simulink model "nonlinear_balsa_v3"  (Simulink 7.8)
settings: Solver=ode45  StartTime=0  StopTime=10  FixedStep=dt_sim  RelTol=1e-6
undefined symbols (not defined in the file): geo, X0
libraries: vrlib x2, dspmtrx3 x1
settings Model: Creator=vickTJ  LastModifiedBy=Dan  BufferReuse=off
settings SolverCC: MaxConsecutiveMinStep=3
settings DataIOCC: ExternalInput=[0 0.571613372420885 7.40569399414751 7.40569021323198 0.00019476436772123 0.000191911234858188]  InitialState=[]  LimitDataPoints=off  MaxDataPoints=5000  SaveState=on  SignalLogging=off  DSMLogging=off  StateSaveName=stout
settings OptimizationCC: InlineParams=on  BufferReuse=off
settings DebuggingCC: UnderspecifiedInitializationDetection=Simplified  SolverPrmCheckMsg=none  FcnCallInpInsideContextMsg=Use local settings  UnconnectedInputMsg=none  UnconnectedOutputMsg=none  InitInArrayFormatMsg=none  SFInvalidInputDataAccessInChartInitDiag=none

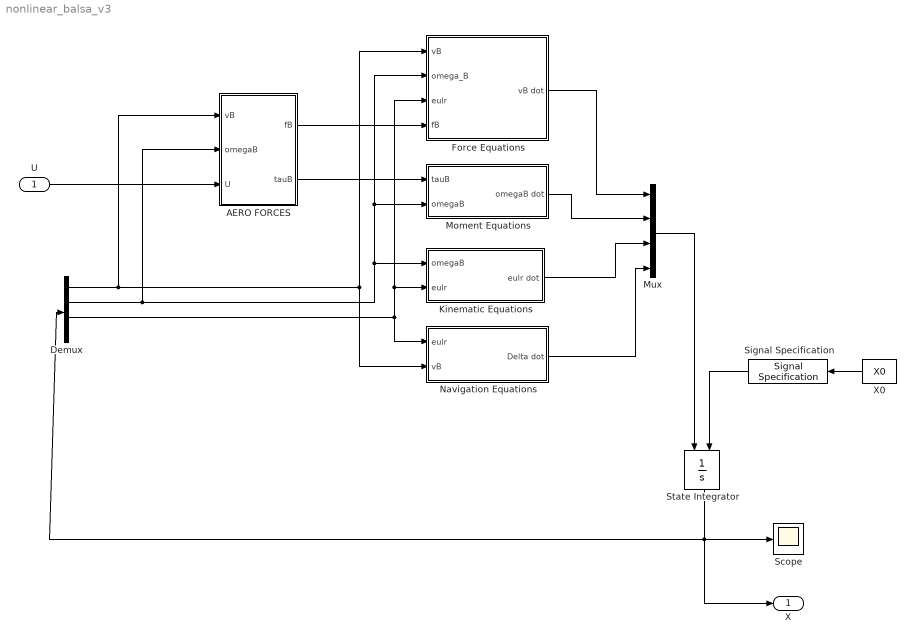
== system nonlinear_balsa_v3 ==
  U : Inport
  AERO FORCES : Subsystem
  Demux : Demux  Outputs=[3,3,3,3]
  Force Equations : Subsystem
  Kinematic Equations : Subsystem
  Moment Equations : Subsystem
  Mux : Mux  Inputs=[3,3,3,3]
  Navigation Equations : Subsystem
  Scope : Scope
  Signal Specification : SignalSpecification  Dimensions=[12,1]
  State Integrator : Integrator  InitialConditionSource=external
  X0 : Constant  Value=X0
  X : Outport
  wires:
  X0/1 -> Signal Specification/1
  Navigation Equations/1(Delta dot) -> Mux/4
  Kinematic Equations/1(eulr dot) -> Mux/3
  Mux/1 -> State Integrator/1
  State Integrator/1 -> Demux/1, Scope/1, X/1
  Force Equations/1(vB dot) -> Mux/1
  Moment Equations/1(omegaB dot) -> Mux/2
  Demux/1 -> Force Equations/1(vB), Navigation Equations/2(vB), AERO FORCES/1(vB)
  Demux/2 -> Force Equations/2(omega_B), Moment Equations/2(omegaB), Kinematic Equations/1(omegaB), AERO FORCES/2(omegaB)
  Demux/3 -> Force Equations/3(eulr), Kinematic Equations/2(eulr), Navigation Equations/1(eulr)
  AERO FORCES/1(fB) -> Force Equations/4(fB)
  AERO FORCES/2(tauB) -> Moment Equations/1(tauB)
  Signal Specification/1 -> State Integrator/2
  U/1 -> AERO FORCES/3(U)

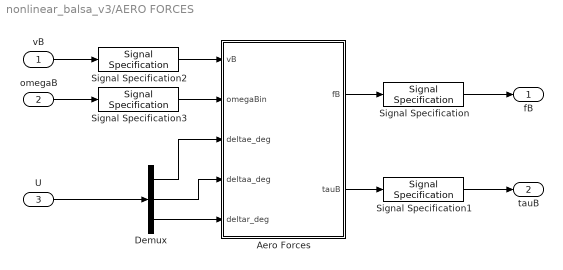
== system nonlinear_balsa_v3/AERO FORCES ==
  vB : Inport
  omegaB : Inport  Port=2
  U : Inport  Port=3
  Aero Forces : MATLAB Function  TreatAsAtomicUnit=on
  Demux : Demux  Outputs=3
  Signal Specification{,1..3} (4 alike) : SignalSpecification  Dimensions=[3,1]
  fB : Outport
  tauB : Outport  Port=2
  wires:
  Aero Forces/1(fB) -> Signal Specification/1
  Aero Forces/2(tauB) -> Signal Specification1/1
  Signal Specification/1 -> fB/1
  Signal Specification1/1 -> tauB/1
  vB/1 -> Signal Specification2/1
  omegaB/1 -> Signal Specification3/1
  Signal Specification2/1 -> Aero Forces/1(vB)
  Signal Specification3/1 -> Aero Forces/2(omegaBin)
  Demux/1 -> Aero Forces/3(deltae_deg)
  Demux/2 -> Aero Forces/4(deltaa_deg)
  Demux/3 -> Aero Forces/5(deltar_deg)
  U/1 -> Demux/1

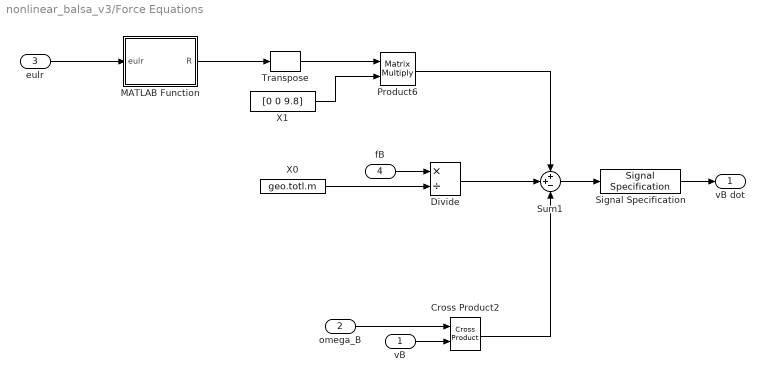
== system nonlinear_balsa_v3/Force Equations ==
  vB : Inport
  omega_B : Inport  Port=2
  eulr : Inport  Port=3
  fB : Inport  Port=4
  Cross Product2 : vrlib/Utilities/Cross Product
  Divide : Product  Inputs=*/
  MATLAB Function : MATLAB Function  TreatAsAtomicUnit=on
  Product6 : Product  Multiplication=Matrix(*)  RndMeth=Zero
  Signal Specification : SignalSpecification  Dimensions=[3,1]
  Sum1 : Sum  Inputs=++-
  Transpose : dspmtrx3/Transpose  Hermitian=off  overflowFlag=off
  X0 : Constant  Value=geo.totl.m
  X1 : Constant  Value=[0 0 9.8]
  vB dot : Outport
  wires:
  omega_B/1 -> Cross Product2/1
  Sum1/1 -> Signal Specification/1
  vB/1 -> Cross Product2/2
  Transpose/1 -> Product6/1
  X1/1 -> Product6/2
  Product6/1 -> Sum1/1
  Cross Product2/1 -> Sum1/3
  Divide/1 -> Sum1/2
  fB/1 -> Divide/1
  X0/1 -> Divide/2
  eulr/1 -> MATLAB Function/1(eulr)
  MATLAB Function/1(R) -> Transpose/1
  Signal Specification/1 -> vB dot/1

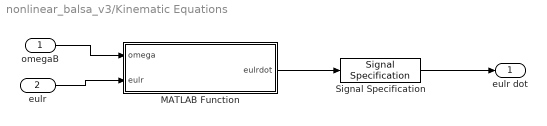
== system nonlinear_balsa_v3/Kinematic Equations ==
  omegaB : Inport
  eulr : Inport  Port=2
  MATLAB Function : MATLAB Function  TreatAsAtomicUnit=on
  Signal Specification : SignalSpecification  Dimensions=[3,1]
  eulr dot : Outport
  wires:
  omegaB/1 -> MATLAB Function/1(omega)
  eulr/1 -> MATLAB Function/2(eulr)
  MATLAB Function/1(eulrdot) -> Signal Specification/1
  Signal Specification/1 -> eulr dot/1

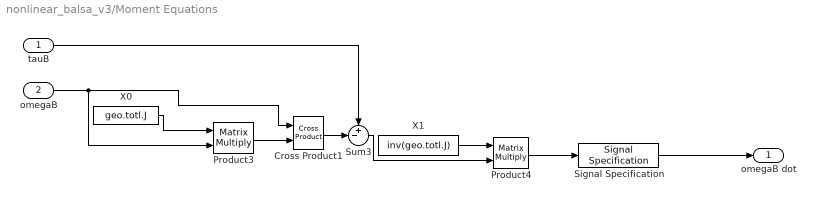
== system nonlinear_balsa_v3/Moment Equations ==
  tauB : Inport
  omegaB : Inport  Port=2
  Cross Product1 : vrlib/Utilities/Cross Product
  Product3 : Product  Multiplication=Matrix(*)  RndMeth=Zero
  Product4 : Product  Multiplication=Matrix(*)  RndMeth=Zero
  Signal Specification : SignalSpecification  Dimensions=[3,1]
  Sum3 : Sum  Inputs=+-|
  X0 : Constant  Value=geo.totl.J
  X1 : Constant  Value=inv(geo.totl.J)
  omegaB dot : Outport
  wires:
  Product4/1 -> Signal Specification/1
  X0/1 -> Product3/1
  omegaB/1 -> Product3/2, Cross Product1/1
  tauB/1 -> Sum3/1
  Cross Product1/1 -> Sum3/2
  Sum3/1 -> Product4/2
  Product3/1 -> Cross Product1/2
  X1/1 -> Product4/1
  Signal Specification/1 -> omegaB dot/1

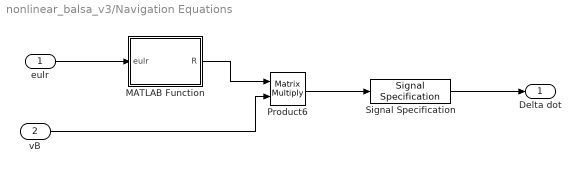
== system nonlinear_balsa_v3/Navigation Equations ==
  eulr : Inport
  vB : Inport  Port=2
  MATLAB Function : MATLAB Function  TreatAsAtomicUnit=on
  Product6 : Product  Multiplication=Matrix(*)  RndMeth=Zero
  Signal Specification : SignalSpecification  Dimensions=[3,1]
  Delta dot : Outport
  wires:
  eulr/1 -> MATLAB Function/1(eulr)
  MATLAB Function/1(R) -> Product6/1
  vB/1 -> Product6/2
  Product6/1 -> Signal Specification/1
  Signal Specification/1 -> Delta dot/1

== matlab function Force Equations/MATLAB Function ==
  data: eulr input double; R output double
function R =eulr2R(eulr)
    phi=eulr(1);
    theta=eulr(2);
    psi=eulr(3);
    R=[cos(psi)*cos(theta), cos(psi)*sin(phi)*sin(theta)-cos(phi)*sin(psi), sin(phi)*sin(psi)+cos(phi)*cos(psi)*sin(theta);
        cos(theta)*sin(psi), cos(phi)*cos(psi)+sin(phi)*sin(psi)*sin(theta), cos(phi)*sin(psi)*sin(theta)-cos(psi)*sin(phi);
        -sin(theta), cos(theta)*sin(phi), cos(phi)*cos(theta)];
end

== matlab function Kinematic Equations/MATLAB Function ==
  data: omega input double; eulr input double; eulrdot output double
function eulrdot=omega2eulrdot(omega,eulr)
    p=omega(1);
    q=omega(2);
    r=omega(3);
    phi=eulr(1);
    theta=eulr(2);
    psi=eulr(3);
    eulrdot=[1 tan(theta)*sin(phi) tan(theta)*cos(phi); 0 cos(phi) -sin(phi); 0 sin(phi)/cos(theta) cos(phi)/cos(theta)]*[p; q; r];
end

== matlab function Navigation Equations/MATLAB Function ==
  data: eulr input double; R output double
function R =eulr2R(eulr)
    phi=eulr(1);
    theta=eulr(2);
    psi=eulr(3);
    R=[cos(psi)*cos(theta), cos(psi)*sin(phi)*sin(theta)-cos(phi)*sin(psi), sin(phi)*sin(psi)+cos(phi)*cos(psi)*sin(theta);
        cos(theta)*sin(psi), cos(phi)*cos(psi)+sin(phi)*sin(psi)*sin(theta), cos(phi)*sin(psi)*sin(theta)-cos(psi)*sin(phi);
        -sin(theta), cos(theta)*sin(phi), cos(phi)*cos(theta)];
end

== matlab function AERO FORCES/Aero Forces ==
  data: fB output double; tauB output double; vB input double; omegaBin input double; deltae_deg input double; deltaa_deg input double; deltar_deg input double
function [fB,tauB]=aero_forces_v1(vB,omegaBin,deltae_deg,deltaa_deg,deltar_deg)

[m,n]=size(omegaBin);
if m==n %if input is square, skew-symmetric matrix: calculate output vector
    omegaB=[0.5*(omegaBin(3,2)-omegaBin(2,3)), 0.5*(-omegaBin(3,1)+omegaBin(1,3)), 0.5*(omegaBin(2,1)-omegaBin(1,2))];
else
    omegaB=[0 -omegaBin(3) omegaBin(2); omegaBin(3) 0 -omegaBin(1); -omegaBin(2) omegaBin(1) 0];

% vB=vB*2;
% omegaB=omegaB*2;
% xihatB=[[0 -0.2948 0.5520; 0.2948 0 0.0009; -0.5520 -0.0009 0] [1; 1; 1]; zeros(1,4)];

xihatB=[omegaB [vB(1); vB(2); vB(3)]; zeros(1,4)];

%%%%%%%%%%%%%%%%%%%%%%%%%%%%%%%%%%%%%%%%%%%%%%%%%%%%%%%%%%%%%%%%%%%%%%%%%%%
%Control surface deflections in radians
aer.delt.e=deltae_deg*pi/180;
aer.delt.a=deltaa_deg*pi/180;
aer.delt.r=deltar_deg*pi/180;

vel.totl=[xihatB(1,4) xihatB(2,4) xihatB(3,4)];
vel.u=vel.totl(1);
vel.v=vel.totl(2);
vel.w=vel.totl(3);
vel.omega=hat(xihatB(1:3,1:3));
vel.p=vel.omega(1);
vel.q=vel.omega(2);
vel.r=vel.omega(3);
vel.VT=norm(vel.totl);
vel.alpha=atan2(vel.w,vel.u); 
vel.beta=asin(vel.v/vel.VT);

%%%%%%%%%%%%%%%%%%%%%%%%%%%%%%%%%%%%%%%%%%%%%%%%%%%%%%%%%%%%%%%%%%%%%%%%%%%
%LONGITUDINAL DYNAMICS
%Calculate effective uvw velocity components at wing (in body axes, NOT including surface deflections)
vel.wing.totl=vel.totl+cross(vel.omega,XYZ.wing.rqc);
vel.wing.u=vel.wing.totl(1);
vel.wing.v=vel.wing.totl(2);
vel.wing.w=vel.wing.totl(3);
vel.wing.VT=norm(vel.wing.totl);
vel.wing.alpha=atan2(vel.wing.w,vel.wing.u); 
vel.wing.beta=asin(vel.wing.v/vel.wing.VT);

%Calculate effective uvw velocity components at horizontal tail (in body axes, including surface deflections)
vel.htai.totl=vel.totl+cross(vel.omega,XYZ.htai.rqc);
vel.htai.u=vel.htai.totl(1);
vel.htai.v=vel.htai.totl(2);
vel.htai.w=vel.htai.totl(3);
vel.htai.VT=norm(vel.htai.totl);
vel.htai.alpha=atan2(vel.htai.w,vel.htai.u)+aer.delt.e; 
vel.htai.beta=asin(vel.htai.v/vel.htai.VT);

%Calculate lift coefficient and total lift force for wing 
aer.wing.CL=(pi*geo.wing.AR*vel.wing.alpha)/(1+sqrt(1+(geo.wing.AR/2)^2));
aer.wing.L=0.5*geo.dens.air*(vel.wing.VT^2)*geo.wing.S*aer.wing.CL;

%Calculate lift coefficient and total lift force for horizontal tail
aer.htai.CL=(pi*geo.htai.AR*(vel.htai.alpha))/(1+sqrt(1+(geo.htai.AR/2)^2));
aer.htai.L=0.5*geo.dens.air*(vel.htai.VT^2)*geo.htai.S*aer.htai.CL;

%Calculate drag coefficient and total drag force for wing 
aer.wing.CD=(aer.wing.CL^2)/(pi*geo.wing.AR*aer.wing.e);
aer.wing.D=0.5*geo.dens.air*(vel.wing.VT^2)*geo.wing.S*aer.wing.CD;

%Calculate drag coefficient and total drag force for horizontal tail
aer.htai.CD=(aer.htai.CL^2)/(pi*geo.htai.AR*aer.htai.e);
aer.htai.D=0.5*geo.dens.air*(vel.htai.VT^2)*geo.htai.S*aer.htai.CD;

%Calculate X components of lift and drag for wing
aer.wing.FXL=aer.wing.L*sin(vel.alpha);
aer.wing.FXD=-aer.wing.D*cos(vel.alpha);

%Calculate X components of lift and drag for horizontal tail
aer.htai.FXL=aer.htai.L*sin(vel.alpha);
aer.htai.FXD=-aer.htai.D*cos(vel.alpha);

%Calculate Z components of lift and drag for wing 
aer.wing.FZL=-aer.wing.L*cos(vel.alpha);
aer.wing.FZD=-aer.wing.D*sin(vel.alpha);

%Calculate Z components of lift and drag for horizontal tail
aer.htai.FZL=-aer.htai.L*cos(vel.alpha);
aer.htai.FZD=-aer.htai.D*sin(vel.alpha);

%Calculate moment MY about Y-axis due to wing and horizontal tail force components FZ_ and FX_
aer.wing.MYL=aer.wing.FZL*XYZ.wing.xdqc+aer.wing.FXL*XYZ.wing.zdcg;
aer.wing.MYD=aer.wing.FZD*XYZ.wing.xdqc+aer.wing.FXD*XYZ.wing.zdcg;
aer.htai.MYL=-aer.htai.FZL*XYZ.htai.xdqc+aer.htai.FXL*XYZ.htai.zdcg;
aer.htai.MYD=-aer.htai.FZD*XYZ.htai.xdqc+aer.htai.FXD*XYZ.htai.zdcg;

%%%%%%%%%%%%%%%%%%%%%%%%%%%%%%%%%%%%%%%%%%%%%%%%%%%%%%%%%%%%%%%%%%%%%%%%%%%
%LATERAL DYNAMICS
%Calculate effective uvw velocity components at vertical tail (in body axes, including surface deflections)
vel.vtai.totl=vel.totl+cross(vel.omega,XYZ.vtai.rqc);
vel.vtai.u=vel.vtai.totl(1);
vel.vtai.v=vel.vtai.totl(2);
vel.vtai.w=vel.vtai.totl(3);
vel.vtai.VT=norm(vel.vtai.totl);
vel.vtai.alpha=asin(vel.vtai.v/vel.vtai.VT)-aer.delt.r; 

%Calculate lift coefficient and lift force for vertical tail
aer.vtai.CL=(pi*geo.vtai.AR*vel.vtai.alpha)/(1+sqrt(1+(geo.vtai.AR/2)^2));
aer.vtai.L=0.5*geo.dens.air*vel.vtai.VT^2*geo.vtai.S*aer.vtai.CL;

%Calculate drag coefficient and drag and drag force for vertical tail
aer.vtai.CD=(aer.vtai.CL^2)/(pi*geo.vtai.AR*aer.vtai.e);
aer.vtai.D=0.5*geo.dens.air*(vel.vtai.VT^2)*geo.vtai.S*aer.vtai.CD;

%Calculate X components of lift and drag for vertical tail
aer.vtai.FXL=aer.vtai.L*sin(vel.vtai.alpha);
aer.vtai.FXD=-aer.vtai.D*cos(vel.vtai.alpha);

%Calculate Y components of lift and drag for vertical tail
aer.vtai.FYL=-aer.vtai.L*cos(vel.vtai.alpha);
aer.vtai.FYD=-aer.vtai.D*cos(vel.vtai.alpha);

% Calculate moment about X-axis: MX
aer.wing.dCL=(pi*geo.wing.AR*aer.delt.a)/(1+sqrt(1+(geo.wing.AR/2)^2));
aer.wing.MX=(0.5*geo.dens.air*vel.wing.VT^2*geo.wing.S*aer.wing.dCL*0.5*geo.wing.b);%*sign(aer.delt.a);

%Calculate moment about Z-axis: MZ
aer.vtai.MZ=aer.vtai.FYL*XYZ.vtai.xdqc+aer.vtai.FYD*XYZ.vtai.xdqc;

%%%%%%%%%%%%%%%%%%%%%%%%%%%%%%%%%%%%%%%%%%%%%%%%%%%%%%%%%%%%%%%%%%%%%%%%%%%
%DAMPING

aer.damp.MX=-0.01*vel.omega(1);
aer.damp.MY=-0.1*vel.omega(2);
aer.damp.MZ=-0.01*vel.omega(3);

%%%%%%%%%%%%%%%%%%%%%%%%%%%%%%%%%%%%%%%%%%%%%%%%%%%%%%%%%%%%%%%%%%%%%%%%%%%
%SUM TOTALS

aer.totl.FX=aer.wing.FXL+aer.wing.FXD+aer.htai.FXL+aer.htai.FXD;
aer.totl.FY=aer.vtai.FYL+aer.vtai.FYD;
aer.totl.FZ=aer.wing.FZL+aer.wing.FZD+aer.htai.FZL+aer.htai.FZD;

aer.totl.MX=aer.wing.MX+aer.damp.MX;
aer.totl.MY=aer.wing.MYL+aer.wing.MYD+aer.htai.MYL+aer.htai.MYD+aer.damp.MY;
aer.totl.MZ=aer.vtai.MZ;

%OUTPUTS
fB=[aer.totl.FX; aer.totl.FY; aer.totl.FZ];
tauB=[aer.totl.MX; aer.totl.MY; aer.totl.MZ];

end
